simulink model "arduino_serial_gps"  (R2024b)
settings: Solver=FixedStepAuto  StartTime=0.0  StopTime=50  RelTol=1e-3  EnableMultiTasking=on
libraries: arduinolib x1
settings Model: SimulationMode=external  ExtModeTrigDuration=2  ExtModeArchiveDirName=C:\Users\mmordeka\Desktop\2_6_morning  ExtModeAddSuffixToVar=on  Creator=The MathWorks, Inc.  LastModifiedBy=Nitesh
settings SolverCC: AlgebraicLoopSolver=TrustRegion  AutoInsertRateTranBlk=on
settings DataIOCC: ReturnWorkspaceOutputs=off
settings OptimizationCC: PassReuseOutputArgsThreshold=0  MaxStackSize=64
settings DebuggingCC: ParameterTunabilityLossMsg=error  UnconnectedInputMsg=warning  UnconnectedOutputMsg=warning  UnconnectedLineMsg=warning  ArithmeticOperatorsInVariantConditions=warning
settings HardwareCC: ProdBitPerPointer=32  ProdBitPerSizeT=32  ProdBitPerPtrDiffT=32  ProdLargestAtomicInteger=Long  ProdLargestAtomicFloat=Double  ProdWordSize=32  ProdHWDeviceType=ARM Compatible->ARM Cortex  UseEmbeddedCoderFeatures=off
settings ModelReferenceCC: EnableRefExpFcnMdlSchedulingChecks=on
settings SFSimCC: SimUseLocalCustomCode=off  MATLABDynamicMemAlloc=off
settings RTWCC: Description=Embedded Coder  SystemTargetFile=ert.tlc  HardwareBoard=ESP32-WROOM(Arduino Compatible)  TLCOptions="-aInlineSetEventsForThisBaseRateFcn=TLC_FALSE -aSuppressMultiTaskScheduler=TLC_FALSE  -aRateBasedStepFcn=0"  TemplateMakefile=ert_default_tmf  GenerateReport=on  RTWUseLocalCustomCode=off  Toolchain=ESP32  BuildConfiguration=Faster Runs  LaunchReport=on  GPUComputeCapability=3.5
settings RTWCC: CustomInitializer=|
  | function addCustomFiles(buildInfo)
  |     % Add GPS Parser Source File
  |     addSourceFiles(buildInfo, {'gps_parser.cpp'}, 'C:/Users/Nitesh/Desktop/exp/GPS_example/src/');
  | 
  |     % Add GPS Parser Header File
  |     addIncludePaths(buildInfo, 'C:/Users/Nitesh/Desktop/exp/GPS_example/src/');
  | 
  |     % Display confirmation message
  |     disp('✅ gps_parser.cpp and header paths added successfully!');
  | end
  | addCustomFiles(buildInfo);
settings CodeAppCC: ForceParamTrailComments=on  OperatorAnnotations=on  StateflowObjectComments=on  MATLABSourceComments=on
settings ERTTargetCC: ERTCustomFileBanners=off  SupportContinuousTime=on  SupportNonInlinedSFcns=on  RemoveResetFunc=off  SupportVariableSizeSignals=on  ModelStepFunctionPrototypeControlCompliant=off  ExtModeTransport=3  ExtModeStaticAlloc=on  ExtModeAutomaticAllocSize=off  ExtModeStaticAllocSize=65536  ExtModeMexFile=ext_xcp  ExtModeIntrfLevel=Level2 - Open  InlinedParameterPlacement=Hierarchical  DynamicArrayContainerType=coder::array

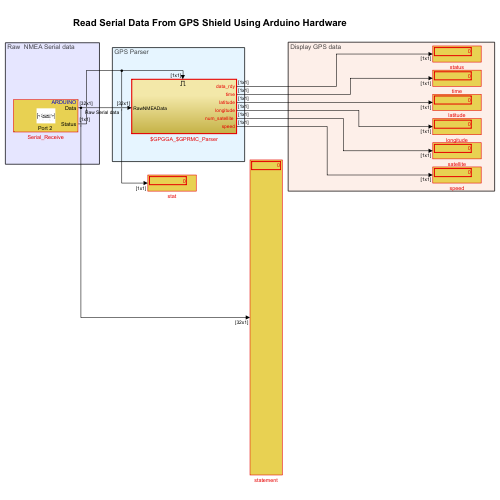
[thumbnail: Simulink's stored preview of the top-level diagram]
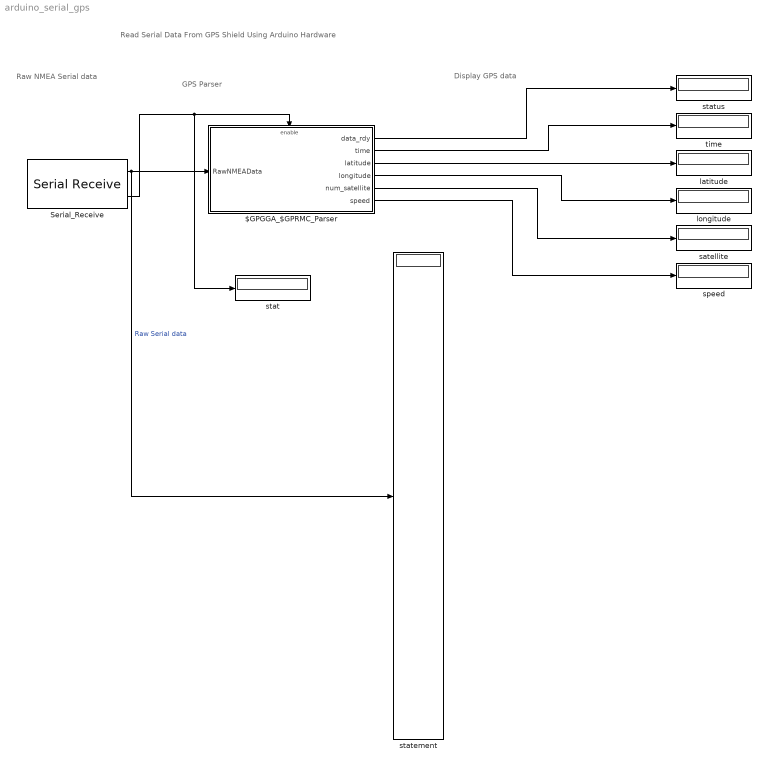
== system arduino_serial_gps ==
  note: Display GPS data
  note: GPS Parser
  note: Raw NMEA Serial data
  note: Read Serial Data From GPS Shield Using Arduino Hardware
  $GPGGA_$GPRMC_Parser : Subsystem  TreatAsAtomicUnit=on
  Serial_Receive : arduinolib/Serial Receive  portNumber=2  DataType=uint8  blockPlatform=arduino  TimeOut=0  MaxDataLength=10  isARMArch=off  DataLengthOption=Length via dialog  Datalength=32  Header=[]  Terminator=[]  SampleTime=0.03  ShowOutStatus=on
      settings: SourceProductName=Common
  latitude : Display
  longitude : Display
  satellite : Display
  speed : Display
  stat : Display
  statement : Display
  status : Display
  time : Display
  wires:
  Serial_Receive/1 -> $GPGGA_$GPRMC_Parser/1(RawNMEAData), statement/1  "Raw Serial data"
  Serial_Receive/2 -> stat/1, $GPGGA_$GPRMC_Parser/Enable
  $GPGGA_$GPRMC_Parser/3(latitude) -> latitude/1
  $GPGGA_$GPRMC_Parser/1(data_rdy) -> status/1
  $GPGGA_$GPRMC_Parser/6(speed) -> speed/1
  $GPGGA_$GPRMC_Parser/2(time) -> time/1
  $GPGGA_$GPRMC_Parser/5("num_satellite ") -> satellite/1
  $GPGGA_$GPRMC_Parser/4(longitude) -> longitude/1

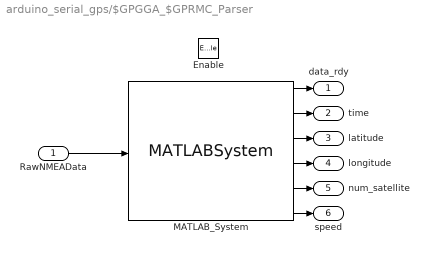
== system arduino_serial_gps/$GPGGA_$GPRMC_Parser ==
  RawNMEAData : Inport
  Enable : EnablePort  StatesWhenEnabling=reset
  MATLAB_System : MATLABSystem  System=GPSParser  TimeOpt=on  LatOpt=on  LonOpt=on  NoSatOpt=on  HdopOpt=off  AltOpt=off  MslOpt=off  SpeedOpt=on  DateOpt=off  TckAngOpt=off
      mask Type: GPSParser
      mask Display:
      | disp('GPSParser');
      | port_label('input',1,'inData');
      | port_label('output',1,'Status');
      | port_label('output',2,'Time');
      | port_label('output',3,'Latitude');
      | port_label('output',4,'Longitude');
      | port_label('output',5,'Satellite');
      | port_label('output',6,'Speed');
  data_rdy : Outport  OutputWhenDisabled=reset  InitialOutput=0  VectorParamsAs1DForOutWhenUnconnected=off
  time : Outport  Port=2  OutputWhenDisabled=reset  InitialOutput=0  VectorParamsAs1DForOutWhenUnconnected=off
  latitude : Outport  Port=3  OutputWhenDisabled=reset  InitialOutput=0  VectorParamsAs1DForOutWhenUnconnected=off
  longitude : Outport  Port=4  OutputWhenDisabled=reset  InitialOutput=0  VectorParamsAs1DForOutWhenUnconnected=off
  "num_satellite " : Outport  Port=5  OutputWhenDisabled=reset  InitialOutput=0  VectorParamsAs1DForOutWhenUnconnected=off
  speed : Outport  Port=6  OutputWhenDisabled=reset  InitialOutput=0  VectorParamsAs1DForOutWhenUnconnected=off
  wires:
  MATLAB_System/1 -> data_rdy/1
  RawNMEAData/1 -> MATLAB_System/1
  MATLAB_System/2 -> time/1
  MATLAB_System/3 -> latitude/1
  MATLAB_System/4 -> longitude/1
  MATLAB_System/5 -> "num_satellite "/1
  MATLAB_System/6 -> speed/1
